simulink model "P_Control"  (R2024b)
settings: Solver=VariableStepAuto  StartTime=0.0  StopTime=time  RelTol=1e-3
values from neighbouring files (symbols this model uses):
  As = 2.15    [Data.m]
  B = (y1-y4)/2    (= 0.75)    [Data.m]
  Cd = 0.28    [Data.m]
  clockwise = 1    [Data.m]
  dd = 2    [Data.m]
  delay_Pulse_time = 1.5    [Data.m]
  derta1 = 0.5    [Data.m]
  dk = 2    [Data.m]
  Fi = Ti/r    (= 156.25)    [Data.m]
  Fz = la/(la+lb)*m*g/2    (= 2450)    [Data.m]
  id = 0.01    [Data.m]
  ik = 1    [Data.m]
  Iw = 0.5    [Data.m]
  Iz = 1600    [Data.m]
  JL = 0.08    [Data.m]
  Jm = 6.96e-6    (= 6.96e-06)    [Data.m]
  Kb = 0.0525    [Data.m]
  Kf = 1.4e-3    (= 0.0014)    [Data.m]
  Km = 0.053    [Data.m]
  L = 6.2e-4    (= 0.00062)    [Data.m]    (also in submit.m = (1-nameda1)*(1-0.015*u1*sqrt((cx^2)*(nameda1^2)+(cy^2)*((tan)
  la = x1    (= 1.25)    [Data.m]
  lb = x1    (= 1.25)    [Data.m]
  m = 1000    [Data.m]
  modeli = 1    [Data.m]
  n = 1/200    (= 0.005)    [Data.m]
  pd = 100    [Data.m]
  pk = 300    [Data.m]
  Pulse = 180    [Data.m]
  R = 2.07    [Data.m]
  r = 0.32    [Data.m]
  s_ang3 = 0    [Data.m]
  x1 = 1.25    [Data.m]
  x1_fc = 0.01    [Data.m]
  x1_jz = 0    [Data.m]
  x2 = -1.25    [Data.m]
  x2_fc = 0.05    [Data.m]
  x2_jz = 0.01    [Data.m]
  x3 = -1.25    [Data.m]
  x3_fc = 0.1    [Data.m]
  x3_jz = 0.05    [Data.m]
  x4 = 1.25    [Data.m]
  x4_fc = 0.5    [Data.m]
  x4_jz = 0.08    [Data.m]
  Xicr = 0,Yicr=10    [Data.m]
  y1 = 0.75    [Data.m]
  y2 = 0.75    [Data.m]
  y3 = -0.75    [Data.m]
  y4 = -0.75    [Data.m]
undefined symbols (not defined in the file or in its folder): Yicr
libraries: slpidlib x12
(part 1 of 2)
settings Model: Creator=hzh  LastModifiedBy=hzh
settings DataIOCC: ReturnWorkspaceOutputsName=out1
settings RTWCC: GPUComputeCapability=3.5

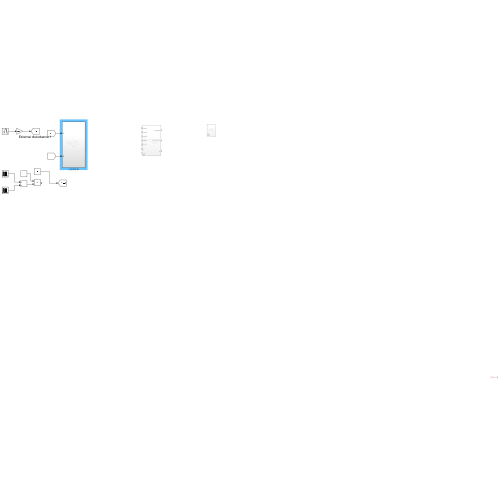
[thumbnail: Simulink's stored preview of the top-level diagram]
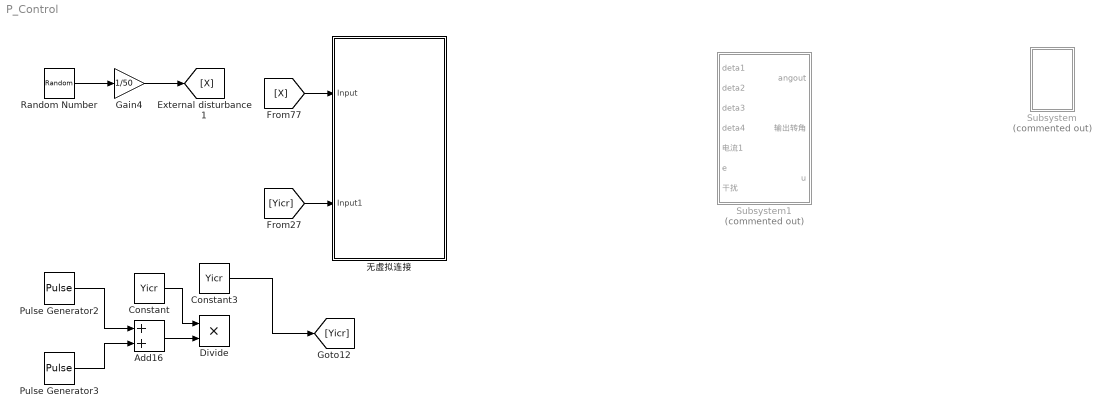
== system P_Control ==
  Add16 : Sum
  Constant : Constant  Value=Yicr
  Constant3 : Constant  Value=Yicr
  Divide : Product  Inputs=**
  Gain4 : Gain  Gain=1/50
  Pulse Generator2 : DiscretePulseGenerator  PulseType=Time based  Period=5  PulseWidth=50
  Pulse Generator3 : DiscretePulseGenerator  PulseType=Time based  Amplitude=-1  Period=5  PulseWidth=50  PhaseDelay=2.5
  Random Number : RandomNumber  SampleTime=0.1
  Subsystem : Subsystem  Commented=on
  Subsystem1 : Subsystem  Commented=on
  无虚拟连接 : Subsystem
  wires:
  ? -> ?
  [Yicr] -> 无虚拟连接/2(Input1)
  [X] -> 无虚拟连接/1(Input)
  Random Number/1 -> Gain4/1
  Gain4/1 -> [X]
  Pulse Generator3/1 -> Add16/2
  Constant/1 -> Divide/1
  Pulse Generator2/1 -> Add16/1
  Add16/1 -> Divide/2
  Constant3/1 -> [Yicr]

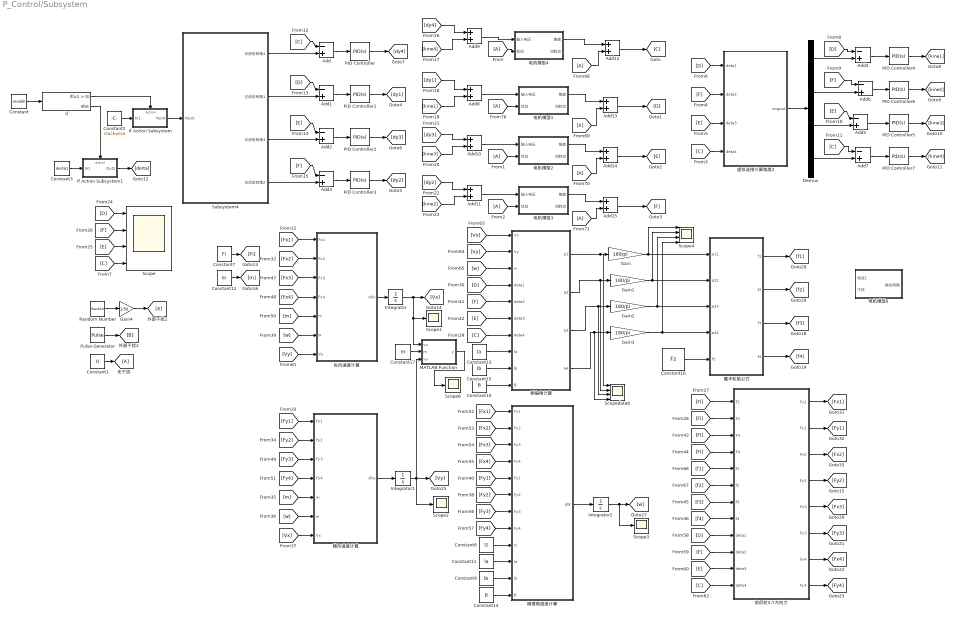
== system P_Control/Subsystem ==
  Add{,1..7} (8 alike) : Sum  Inputs=-+
  Add{8..15} (8 alike) : Sum
  Constant : Constant  Value=modeli
  Constant1 : Constant  Value=0
  Constant10 : Constant  Value=B
  Constant11 : Constant  Value=la
  Constant12 : Constant  Value=m
  Constant13 : Constant  Value=la
  Constant14 : Constant  Value=B
  Constant15 : Constant  Value=lb
  Constant16 : Constant  Value=Fz
  Constant17 : Constant  Value=m
  Constant2 : Constant  Value=clockwise
  Constant3 : Constant  Value=derta1
  Constant7 : Constant  Value=Fi
  Constant8 : Constant  Value=Iz
  Constant9 : Constant  Value=lb
  Demux : Demux
  From{,1..2,68,70..71,76} (7 alike) : From
  Gain{,1..3} (4 alike) : Gain  Gain=180/pi
  Gain4 : Gain  Gain=1/50
  If : If
  If Action Subsystem : Subsystem  TreatAsAtomicUnit=on
  If Action Subsystem1 : Subsystem  TreatAsAtomicUnit=on
  Integrator : Integrator  InitialCondition=0.01
  Integrator1 : Integrator
  Integrator2 : Integrator
  MATLAB Function : MATLAB Function  TreatAsAtomicUnit=on
  PID Controller{,1..3} (4 alike) : slpidlib/PID Controller  Controller=PID  Form=Parallel  TimeDomain=Continuous-time  UseExternalTs=off  SampleTime=-1  IntegratorMethod=Forward Euler  FilterMethod=Forward Euler  ControllerParametersSource=internal  P=pd  I=id  UseKiTs=off  D=dd  N=100  UseFilter=on  TunerSelectOption=Transfer Function Based (PID Tuner App)  InitialConditionSource=internal  InitialConditionForIntegrator=0  InitialConditionForFilter=0  DifferentiatorICPrevScaledInput=0  ExternalReset=none  TrackingMode=off  Kt=1  LimitOutput=off  SatLimitsSource=internal  UpperSaturationLimit=inf  LowerSaturationLimit=-inf  LinearizeAsGain=on  AntiWindupMode=none  Kb=1  LimitIntegrator=off  UpperIntegratorSaturationLimit=inf  LowerIntegratorSaturationLimit=-inf  POutMin=[]  POutMax=[]  IOutMin=[]  IOutMax=[]  DOutMin=[]  DOutMax=[]  NOutMin=[]  NOutMax=[]  SumOutMin=[]  SumOutMax=[]  SaturationOutMin=[]  SaturationOutMax=[]  PParamMin=[]  PParamMax=[]  IParamMin=[]  IParamMax=[]  DParamMin=[]  DParamMax=[]  NParamMin=[]  NParamMax=[]  KbParamMin=[]  KbParamMax=[]  KtParamMin=[]  KtParamMax=[]  KbOutMin=[]  KbOutMax=[]  KtOutMin=[]  KtOutMax=[]  IntegratorOutMin=[]  IntegratorOutMax=[]  FilterOutMin=[]  FilterOutMax=[]  SumI1OutMin=[]  SumI1OutMax=[]  SumI2OutMin=[]  SumI2OutMax=[]  SumI3OutMin=[]  SumI3OutMax=[]  SumI4OutMin=[]  SumI4OutMax=[]  SumDOutMin=[]  SumDOutMax=[]  DifferentiatorOutMin=[]  DifferentiatorOutMax=[]  FilterDiffOutCoefMin=[]  FilterDiffOutCoefMax=[]  ReciprocalOutMin=[]  ReciprocalOutMax=[]  SumDenOutMin=[]  SumDenOutMax=[]  SumNumOutMin=[]  SumNumOutMax=[]  DivideOutMin=[]  DivideOutMax=[]  UdiffTsProdOutMin=[]  UdiffTsProdOutMax=[]  NTsProdOutMin=[]  NTsProdOutMax=[]  UintegralTsProdOutMin=[]  UintegralTsProdOutMax=[]  UngainTsProdOutMin=[]  UngainTsProdOutMax=[]  ClampingZeroOutDataTypeStr=Inherit: Inherit via back propagation  ClampingZeroOutMin=[]  ClampingZeroOutMax=[]  FilterDenConstantOutDataTypeStr=Inherit: Inherit via back propagation  FilterDenConstantOutMin=[]  FilterDenConstantOutMax=[]  PCopyOutDataTypeStr=Inherit: Inherit via back propagation  PCopyOutMin=[]  PCopyOutMax=[]  NCopyOutDataTypeStr=Inherit: Inherit via back propagation  NCopyOutMin=[]  NCopyOutMax=[]  IntegratorContinuousStateAttributes=''  IntegratorStateMustResolveToSignalObject=off  IntegratorRTWStateStorageClass=Auto  FilterContinuousStateAttributes=''  FilterStateMustResolveToSignalObject=off  FilterRTWStateStorageClass=Auto  ParallelPVariant=InternalParameters  IdealPVariant=Disabled  IVariant=InternalParameters  DVariant=InternalParameters  IntegratorVariant=Continuous  SatVariant=Disabled  AWVariant=Passthrough  PCopyVariant=Disabled  TRVariant=Disabled  FdbkBlocksVariant=Forward  IdealPFdbkVariant=Disabled  SatFdbkVariant=Disabled  DerivativeFilterVariant=ContFilter  NVariant=InternalParameters  NCopyVariant=Disabled  FilterICVariant=InternalICsFilter  IntegratorICVariant=InternalICs  ExternalResetVariant=Disabled  TRSumVariant=Passthrough  SumFdbkVariant=Disabled  SumVariant=Sum_PID  TsampFilterVariant=InternalTs  TsampNgainVariant=Passthrough  TsampIntegralVariant=Disabled_SignalSpec  ExternalSaturationOutDataTypeStr=Inherit: Same as second input
  PID Controller4 : slpidlib/PID Controller  Controller=PID  Form=Parallel  TimeDomain=Continuous-time  UseExternalTs=off  SampleTime=-1  IntegratorMethod=Forward Euler  FilterMethod=Forward Euler  ControllerParametersSource=internal  P=pk  I=ik  UseKiTs=off  D=dk  N=100  UseFilter=on  TunerSelectOption=Transfer Function Based (PID Tuner App)  InitialConditionSource=internal  InitialConditionForIntegrator=0  InitialConditionForFilter=0  DifferentiatorICPrevScaledInput=0  ExternalReset=none  TrackingMode=off  Kt=1  LimitOutput=off  SatLimitsSource=internal  UpperSaturationLimit=inf  LowerSaturationLimit=-inf  LinearizeAsGain=on  AntiWindupMode=none  Kb=1  LimitIntegrator=off  UpperIntegratorSaturationLimit=inf  LowerIntegratorSaturationLimit=-inf  POutMin=[]  POutMax=[]  IOutMin=[]  IOutMax=[]  DOutMin=[]  DOutMax=[]  NOutMin=[]  NOutMax=[]  SumOutMin=[]  SumOutMax=[]  SaturationOutMin=[]  SaturationOutMax=[]  PParamMin=[]  PParamMax=[]  IParamMin=[]  IParamMax=[]  DParamMin=[]  DParamMax=[]  NParamMin=[]  NParamMax=[]  KbParamMin=[]  KbParamMax=[]  KtParamMin=[]  KtParamMax=[]  KbOutMin=[]  KbOutMax=[]  KtOutMin=[]  KtOutMax=[]  IntegratorOutMin=[]  IntegratorOutMax=[]  FilterOutMin=[]  FilterOutMax=[]  SumI1OutMin=[]  SumI1OutMax=[]  SumI2OutMin=[]  SumI2OutMax=[]  SumI3OutMin=[]  SumI3OutMax=[]  SumI4OutMin=[]  SumI4OutMax=[]  SumDOutMin=[]  SumDOutMax=[]  DifferentiatorOutMin=[]  DifferentiatorOutMax=[]  FilterDiffOutCoefMin=[]  FilterDiffOutCoefMax=[]  ReciprocalOutMin=[]  ReciprocalOutMax=[]  SumDenOutMin=[]  SumDenOutMax=[]  SumNumOutMin=[]  SumNumOutMax=[]  DivideOutMin=[]  DivideOutMax=[]  UdiffTsProdOutMin=[]  UdiffTsProdOutMax=[]  NTsProdOutMin=[]  NTsProdOutMax=[]  UintegralTsProdOutMin=[]  UintegralTsProdOutMax=[]  UngainTsProdOutMin=[]  UngainTsProdOutMax=[]  ClampingZeroOutDataTypeStr=Inherit: Inherit via back propagation  ClampingZeroOutMin=[]  ClampingZeroOutMax=[]  FilterDenConstantOutDataTypeStr=Inherit: Inherit via back propagation  FilterDenConstantOutMin=[]  FilterDenConstantOutMax=[]  PCopyOutDataTypeStr=Inherit: Inherit via back propagation  PCopyOutMin=[]  PCopyOutMax=[]  NCopyOutDataTypeStr=Inherit: Inherit via back propagation  NCopyOutMin=[]  NCopyOutMax=[]  IntegratorContinuousStateAttributes=''  IntegratorStateMustResolveToSignalObject=off  IntegratorRTWStateStorageClass=Auto  FilterContinuousStateAttributes=''  FilterStateMustResolveToSignalObject=off  FilterRTWStateStorageClass=Auto  ParallelPVariant=InternalParameters  IdealPVariant=Disabled  IVariant=InternalParameters  DVariant=InternalParameters  IntegratorVariant=Continuous  SatVariant=Disabled  AWVariant=Passthrough  PCopyVariant=Disabled  TRVariant=Disabled  FdbkBlocksVariant=Forward  IdealPFdbkVariant=Disabled  SatFdbkVariant=Disabled  DerivativeFilterVariant=ContFilter  NVariant=InternalParameters  NCopyVariant=Disabled  FilterICVariant=InternalICsFilter  IntegratorICVariant=InternalICs  ExternalResetVariant=Disabled  TRSumVariant=Passthrough  SumFdbkVariant=Disabled  SumVariant=Sum_PID  TsampFilterVariant=InternalTs  TsampNgainVariant=Passthrough  TsampIntegralVariant=Disabled_SignalSpec  ExternalSaturationOutDataTypeStr=Inherit: Same as second input
  PID Controller5 : slpidlib/PID Controller  Controller=PID  Form=Parallel  TimeDomain=Continuous-time  UseExternalTs=off  SampleTime=-1  IntegratorMethod=Forward Euler  FilterMethod=Forward Euler  ControllerParametersSource=internal  P=pk  I=ik  UseKiTs=off  D=dk  N=100  UseFilter=on  TunerSelectOption=Frequency Response Based  InitialConditionSource=internal  InitialConditionForIntegrator=0  InitialConditionForFilter=0  DifferentiatorICPrevScaledInput=0  ExternalReset=none  TrackingMode=off  Kt=1  LimitOutput=off  SatLimitsSource=internal  UpperSaturationLimit=inf  LowerSaturationLimit=-inf  LinearizeAsGain=on  AntiWindupMode=none  Kb=1  LimitIntegrator=off  UpperIntegratorSaturationLimit=inf  LowerIntegratorSaturationLimit=-inf  POutMin=[]  POutMax=[]  IOutMin=[]  IOutMax=[]  DOutMin=[]  DOutMax=[]  NOutMin=[]  NOutMax=[]  SumOutMin=[]  SumOutMax=[]  SaturationOutMin=[]  SaturationOutMax=[]  PParamMin=[]  PParamMax=[]  IParamMin=[]  IParamMax=[]  DParamMin=[]  DParamMax=[]  NParamMin=[]  NParamMax=[]  KbParamMin=[]  KbParamMax=[]  KtParamMin=[]  KtParamMax=[]  KbOutMin=[]  KbOutMax=[]  KtOutMin=[]  KtOutMax=[]  IntegratorOutMin=[]  IntegratorOutMax=[]  FilterOutMin=[]  FilterOutMax=[]  SumI1OutMin=[]  SumI1OutMax=[]  SumI2OutMin=[]  SumI2OutMax=[]  SumI3OutMin=[]  SumI3OutMax=[]  SumI4OutMin=[]  SumI4OutMax=[]  SumDOutMin=[]  SumDOutMax=[]  DifferentiatorOutMin=[]  DifferentiatorOutMax=[]  FilterDiffOutCoefMin=[]  FilterDiffOutCoefMax=[]  ReciprocalOutMin=[]  ReciprocalOutMax=[]  SumDenOutMin=[]  SumDenOutMax=[]  SumNumOutMin=[]  SumNumOutMax=[]  DivideOutMin=[]  DivideOutMax=[]  UdiffTsProdOutMin=[]  UdiffTsProdOutMax=[]  NTsProdOutMin=[]  NTsProdOutMax=[]  UintegralTsProdOutMin=[]  UintegralTsProdOutMax=[]  UngainTsProdOutMin=[]  UngainTsProdOutMax=[]  ClampingZeroOutDataTypeStr=Inherit: Inherit via back propagation  ClampingZeroOutMin=[]  ClampingZeroOutMax=[]  FilterDenConstantOutDataTypeStr=Inherit: Inherit via back propagation  FilterDenConstantOutMin=[]  FilterDenConstantOutMax=[]  PCopyOutDataTypeStr=Inherit: Inherit via back propagation  PCopyOutMin=[]  PCopyOutMax=[]  NCopyOutDataTypeStr=Inherit: Inherit via back propagation  NCopyOutMin=[]  NCopyOutMax=[]  IntegratorContinuousStateAttributes=''  IntegratorStateMustResolveToSignalObject=off  IntegratorRTWStateStorageClass=Auto  FilterContinuousStateAttributes=''  FilterStateMustResolveToSignalObject=off  FilterRTWStateStorageClass=Auto  ParallelPVariant=InternalParameters  IdealPVariant=Disabled  IVariant=InternalParameters  DVariant=InternalParameters  IntegratorVariant=Continuous  SatVariant=Disabled  AWVariant=Passthrough  PCopyVariant=Disabled  TRVariant=Disabled  FdbkBlocksVariant=Forward  IdealPFdbkVariant=Disabled  SatFdbkVariant=Disabled  DerivativeFilterVariant=ContFilter  NVariant=InternalParameters  NCopyVariant=Disabled  FilterICVariant=InternalICsFilter  IntegratorICVariant=InternalICs  ExternalResetVariant=Disabled  TRSumVariant=Passthrough  SumFdbkVariant=Disabled  SumVariant=Sum_PID  TsampFilterVariant=InternalTs  TsampNgainVariant=Passthrough  TsampIntegralVariant=Disabled_SignalSpec  ExternalSaturationOutDataTypeStr=Inherit: Same as second input
  PID Controller6 : slpidlib/PID Controller  Controller=PID  Form=Parallel  TimeDomain=Continuous-time  UseExternalTs=off  SampleTime=-1  IntegratorMethod=Forward Euler  FilterMethod=Forward Euler  ControllerParametersSource=internal  P=pk  I=ik  UseKiTs=off  D=dk  N=100  UseFilter=on  TunerSelectOption=Transfer Function Based (PID Tuner App)  InitialConditionSource=internal  InitialConditionForIntegrator=0  InitialConditionForFilter=0  DifferentiatorICPrevScaledInput=0  ExternalReset=none  TrackingMode=off  Kt=1  LimitOutput=off  SatLimitsSource=internal  UpperSaturationLimit=inf  LowerSaturationLimit=-inf  LinearizeAsGain=on  AntiWindupMode=none  Kb=1  LimitIntegrator=off  UpperIntegratorSaturationLimit=inf  LowerIntegratorSaturationLimit=-inf  POutMin=[]  POutMax=[]  IOutMin=[]  IOutMax=[]  DOutMin=[]  DOutMax=[]  NOutMin=[]  NOutMax=[]  SumOutMin=[]  SumOutMax=[]  SaturationOutMin=[]  SaturationOutMax=[]  PParamMin=[]  PParamMax=[]  IParamMin=[]  IParamMax=[]  DParamMin=[]  DParamMax=[]  NParamMin=[]  NParamMax=[]  KbParamMin=[]  KbParamMax=[]  KtParamMin=[]  KtParamMax=[]  KbOutMin=[]  KbOutMax=[]  KtOutMin=[]  KtOutMax=[]  IntegratorOutMin=[]  IntegratorOutMax=[]  FilterOutMin=[]  FilterOutMax=[]  SumI1OutMin=[]  SumI1OutMax=[]  SumI2OutMin=[]  SumI2OutMax=[]  SumI3OutMin=[]  SumI3OutMax=[]  SumI4OutMin=[]  SumI4OutMax=[]  SumDOutMin=[]  SumDOutMax=[]  DifferentiatorOutMin=[]  DifferentiatorOutMax=[]  FilterDiffOutCoefMin=[]  FilterDiffOutCoefMax=[]  ReciprocalOutMin=[]  ReciprocalOutMax=[]  SumDenOutMin=[]  SumDenOutMax=[]  SumNumOutMin=[]  SumNumOutMax=[]  DivideOutMin=[]  DivideOutMax=[]  UdiffTsProdOutMin=[]  UdiffTsProdOutMax=[]  NTsProdOutMin=[]  NTsProdOutMax=[]  UintegralTsProdOutMin=[]  UintegralTsProdOutMax=[]  UngainTsProdOutMin=[]  UngainTsProdOutMax=[]  ClampingZeroOutDataTypeStr=Inherit: Inherit via back propagation  ClampingZeroOutMin=[]  ClampingZeroOutMax=[]  FilterDenConstantOutDataTypeStr=Inherit: Inherit via back propagation  FilterDenConstantOutMin=[]  FilterDenConstantOutMax=[]  PCopyOutDataTypeStr=Inherit: Inherit via back propagation  PCopyOutMin=[]  PCopyOutMax=[]  NCopyOutDataTypeStr=Inherit: Inherit via back propagation  NCopyOutMin=[]  NCopyOutMax=[]  IntegratorContinuousStateAttributes=''  IntegratorStateMustResolveToSignalObject=off  IntegratorRTWStateStorageClass=Auto  FilterContinuousStateAttributes=''  FilterStateMustResolveToSignalObject=off  FilterRTWStateStorageClass=Auto  ParallelPVariant=InternalParameters  IdealPVariant=Disabled  IVariant=InternalParameters  DVariant=InternalParameters  IntegratorVariant=Continuous  SatVariant=Disabled  AWVariant=Passthrough  PCopyVariant=Disabled  TRVariant=Disabled  FdbkBlocksVariant=Forward  IdealPFdbkVariant=Disabled  SatFdbkVariant=Disabled  DerivativeFilterVariant=ContFilter  NVariant=InternalParameters  NCopyVariant=Disabled  FilterICVariant=InternalICsFilter  IntegratorICVariant=InternalICs  ExternalResetVariant=Disabled  TRSumVariant=Passthrough  SumFdbkVariant=Disabled  SumVariant=Sum_PID  TsampFilterVariant=InternalTs  TsampNgainVariant=Passthrough  TsampIntegralVariant=Disabled_SignalSpec  ExternalSaturationOutDataTypeStr=Inherit: Same as second input
  PID Controller7 : slpidlib/PID Controller  Controller=PID  Form=Parallel  TimeDomain=Continuous-time  UseExternalTs=off  SampleTime=-1  IntegratorMethod=Forward Euler  FilterMethod=Forward Euler  ControllerParametersSource=internal  P=pk  I=ik  UseKiTs=off  D=dk  N=100  UseFilter=on  TunerSelectOption=Transfer Function Based (PID Tuner App)  InitialConditionSource=internal  InitialConditionForIntegrator=0  InitialConditionForFilter=0  DifferentiatorICPrevScaledInput=0  ExternalReset=none  TrackingMode=off  Kt=1  LimitOutput=off  SatLimitsSource=internal  UpperSaturationLimit=inf  LowerSaturationLimit=-inf  LinearizeAsGain=on  AntiWindupMode=none  Kb=1  LimitIntegrator=off  UpperIntegratorSaturationLimit=inf  LowerIntegratorSaturationLimit=-inf  POutMin=[]  POutMax=[]  IOutMin=[]  IOutMax=[]  DOutMin=[]  DOutMax=[]  NOutMin=[]  NOutMax=[]  SumOutMin=[]  SumOutMax=[]  SaturationOutMin=[]  SaturationOutMax=[]  PParamMin=[]  PParamMax=[]  IParamMin=[]  IParamMax=[]  DParamMin=[]  DParamMax=[]  NParamMin=[]  NParamMax=[]  KbParamMin=[]  KbParamMax=[]  KtParamMin=[]  KtParamMax=[]  KbOutMin=[]  KbOutMax=[]  KtOutMin=[]  KtOutMax=[]  IntegratorOutMin=[]  IntegratorOutMax=[]  FilterOutMin=[]  FilterOutMax=[]  SumI1OutMin=[]  SumI1OutMax=[]  SumI2OutMin=[]  SumI2OutMax=[]  SumI3OutMin=[]  SumI3OutMax=[]  SumI4OutMin=[]  SumI4OutMax=[]  SumDOutMin=[]  SumDOutMax=[]  DifferentiatorOutMin=[]  DifferentiatorOutMax=[]  FilterDiffOutCoefMin=[]  FilterDiffOutCoefMax=[]  ReciprocalOutMin=[]  ReciprocalOutMax=[]  SumDenOutMin=[]  SumDenOutMax=[]  SumNumOutMin=[]  SumNumOutMax=[]  DivideOutMin=[]  DivideOutMax=[]  UdiffTsProdOutMin=[]  UdiffTsProdOutMax=[]  NTsProdOutMin=[]  NTsProdOutMax=[]  UintegralTsProdOutMin=[]  UintegralTsProdOutMax=[]  UngainTsProdOutMin=[]  UngainTsProdOutMax=[]  ClampingZeroOutDataTypeStr=Inherit: Inherit via back propagation  ClampingZeroOutMin=[]  ClampingZeroOutMax=[]  FilterDenConstantOutDataTypeStr=Inherit: Inherit via back propagation  FilterDenConstantOutMin=[]  FilterDenConstantOutMax=[]  PCopyOutDataTypeStr=Inherit: Inherit via back propagation  PCopyOutMin=[]  PCopyOutMax=[]  NCopyOutDataTypeStr=Inherit: Inherit via back propagation  NCopyOutMin=[]  NCopyOutMax=[]  IntegratorContinuousStateAttributes=''  IntegratorStateMustResolveToSignalObject=off  IntegratorRTWStateStorageClass=Auto  FilterContinuousStateAttributes=''  FilterStateMustResolveToSignalObject=off  FilterRTWStateStorageClass=Auto  ParallelPVariant=InternalParameters  IdealPVariant=Disabled  IVariant=InternalParameters  DVariant=InternalParameters  IntegratorVariant=Continuous  SatVariant=Disabled  AWVariant=Passthrough  PCopyVariant=Disabled  TRVariant=Disabled  FdbkBlocksVariant=Forward  IdealPFdbkVariant=Disabled  SatFdbkVariant=Disabled  DerivativeFilterVariant=ContFilter  NVariant=InternalParameters  NCopyVariant=Disabled  FilterICVariant=InternalICsFilter  IntegratorICVariant=InternalICs  ExternalResetVariant=Disabled  TRSumVariant=Passthrough  SumFdbkVariant=Disabled  SumVariant=Sum_PID  TsampFilterVariant=InternalTs  TsampNgainVariant=Passthrough  TsampIntegralVariant=Disabled_SignalSpec  ExternalSaturationOutDataTypeStr=Inherit: Same as second input
  Pulse Generator : DiscretePulseGenerator  PulseType=Time based  Amplitude=Pulse  Period=100  PulseWidth=0.2  PhaseDelay=delay_Pulse_time
  Random Number : RandomNumber  SampleTime=0.1
  Scope : Scope  NumInputPorts=4
  Scope{1..3,6} (4 alike) : Scope
  Scope4 : Scope  NumInputPorts=4
  Scopedata6 : Scope  NumInputPorts=4
  Subsystem4 : Subsystem
  侧偏角计算 : MATLAB Function  TreatAsAtomicUnit=on
  前后轮X,Y方向力 : MATLAB Function  TreatAsAtomicUnit=on
  无干扰 : Goto
  横向速度计算 : MATLAB Function  TreatAsAtomicUnit=on
  横摆角速度计算 : MATLAB Function  TreatAsAtomicUnit=on
  电机模型1 : Subsystem
  电机模型2 : Subsystem
  电机模型3 : Subsystem
  电机模型4 : Subsystem
  电机模型6 : Subsystem
  纵向速度计算 : MATLAB Function  TreatAsAtomicUnit=on
  虚拟连接计算角度2 : MATLAB Function  TreatAsAtomicUnit=on
  魔术轮胎公式 : MATLAB Function  TreatAsAtomicUnit=on
  wires:
  [C] -> 前后轮X,Y方向力/12(deta4)
  Add2/1 -> PID Controller2/1
  MATLAB Function/1(y) -> Scope6/1
  前后轮X,Y方向力/2(Fy1) -> [Fy1]
  Add12/1 -> [C]
  [w] -> 横向速度计算/6(w)
  [D] -> 侧偏角计算/4(deta1)
  Integrator/1 -> [Vx], MATLAB Function/1(vx), Scope1/1
  PID Controller/1 -> [dy4]
  虚拟连接计算角度2/1(angout) -> Demux/1
  [Fy4] -> 横向速度计算/4(Fy4)
  [Fx1] -> 横摆角速度计算/1(Fx1)
  [m] -> 横向速度计算/5(m)
  [kine4] -> Add9/2
  Add6/1 -> PID Controller6/1
  PID Controller4/1 -> [kine1]
  Add14/1 -> [E]
  前后轮X,Y方向力/3(Fx2) -> [Fx2]
  [f2] -> 前后轮X,Y方向力/6(f2)
  If/1 -> If Action Subsystem/Action
  Gain4/1 -> [X]
  Add11/1 -> 电机模型3/1(输入电压)
  [Fx4] -> 横摆角速度计算/4(Fx4)
  [Fx2] -> 纵向速度计算/2(Fx2)
  Constant16/1 -> 魔术轮胎公式/5(Fz)
  PID Controller2/1 -> [dy3]
  From2/1 -> 电机模型3/2(扰动)
  Demux/2 -> Add6/2
  If/2 -> If Action Subsystem1/Action
  From76/1 -> 电机模型1/2(扰动)
  [Fy2] -> 横向速度计算/2(Fy2)
  Random Number/1 -> Gain4/1
  [Vy] -> 侧偏角计算/2(Vy)
  Gain3/1 -> Scope4/4, 魔术轮胎公式/4(a44)
  [m] -> 纵向速度计算/5(m)
  If Action Subsystem1/1(Out1) -> [derta]
  Constant2/1 -> If Action Subsystem/1(In1)
  Constant12/1 -> [m]
  魔术轮胎公式/1(f1) -> [f1]
  From71/1 -> Add15/2
  Add15/1 -> [F]
  If Action Subsystem/1(Input) -> Subsystem4/1(Input)
  [D] -> 前后轮X,Y方向力/9(deta1)
  Add1/1 -> PID Controller1/1
  PID Controller6/1 -> [kine2]
  PID Controller3/1 -> [dy2]
  [w] -> 侧偏角计算/3(w)
  [E] -> 侧偏角计算/6(deta3)
  Constant10/1 -> 侧偏角计算/10(B)
  From1/1 -> 电机模型2/2(扰动)
  [Fy1] -> 横向速度计算/1(Fy1)
  Add10/1 -> 电机模型2/1(输入电压)
  [C] -> 侧偏角计算/7(deta4)
  Subsystem4/4(左后轮转角2) -> Add3/2
  [F] -> 虚拟连接计算角度2/2(deta2)
  [C] -> 虚拟连接计算角度2/4(deta4)
  魔术轮胎公式/2(f2) -> [f2]
  Subsystem4/3(右后轮转角3) -> Add2/2
  Integrator2/1 -> Scope3/1, [w]
  纵向速度计算/1(dVx) -> Integrator/1
  魔术轮胎公式/4(f4) -> [f4]
  [Fi] -> 前后轮X,Y方向力/1(F1)
  [Fi] -> 前后轮X,Y方向力/3(F3)
  [dy2] -> Add11/1
  Demux/1 -> Add4/2
  [C] -> Add/1
  横摆角速度计算/1(dW) -> Integrator2/1
  Demux/3 -> Add5/2
  [X] -> Add13/2
  Add13/1 -> [D]
  Subsystem4/2(左前轮转角1) -> Add1/2
  From68/1 -> Add12/2
  Subsystem4/1(右前轮转角4) -> Add/2
  Constant1/1 -> 无干扰/1
  [dy4] -> Add9/1
  [dy1] -> Add8/1
  From70/1 -> Add14/2
  Add5/1 -> PID Controller5/1
  PID Controller5/1 -> [kine3]
  [D] -> Scope/1
  Add7/1 -> PID Controller7/1
  Add3/1 -> PID Controller3/1
  [F] -> Add3/1
  [E] -> Add2/1
  [E] -> 虚拟连接计算角度2/3(deta3)
  [D] -> Add1/1
  PID Controller1/1 -> [dy1]
  [D] -> Add4/1
  Constant17/1 -> MATLAB Function/2(m)
  Add/1 -> PID Controller/1
  [Fx3] -> 纵向速度计算/3(Fx3)
  [kine3] -> Add10/2
  侧偏角计算/4(a4) -> Scopedata6/4, Gain3/1
  Constant11/1 -> 横摆角速度计算/10(la)
  Add4/1 -> PID Controller4/1
  侧偏角计算/3(a3) -> Scopedata6/3, Gain2/1
  [Fy4] -> 横摆角速度计算/8(Fy4)
  [E] -> 前后轮X,Y方向力/11(deta3)
  Integrator1/1 -> MATLAB Function/3(vy), Scope2/1, [Vy]
  [E] -> Add5/1
  前后轮X,Y方向力/5(Fx3) -> [Fx3]
  前后轮X,Y方向力/4(Fy2) -> [Fy2]
  Gain1/1 -> Scope4/2, 魔术轮胎公式/2(a22)
  Constant9/1 -> 横摆角速度计算/11(lb)
  [f1] -> 前后轮X,Y方向力/5(f1)
  [dy3] -> Add10/1
  [Fx3] -> 横摆角速度计算/3(Fx3)
  前后轮X,Y方向力/7(Fx4) -> [Fx4]
  Demux/4 -> Add7/2
  Constant13/1 -> 侧偏角计算/8(la)
  [Fy1] -> 横摆角速度计算/5(Fy1)
  [kine1] -> Add8/2
  Constant/1 -> If/1
  侧偏角计算/2(a2) -> Scopedata6/2, Gain1/1
  [w] -> 纵向速度计算/6(w)
  [Fx2] -> 横摆角速度计算/2(Fx2)
  [Fy2] -> 横摆角速度计算/6(Fy2)
  前后轮X,Y方向力/1(Fx1) -> [Fx1]
  Constant15/1 -> 侧偏角计算/9(lb)
  侧偏角计算/1(a1) -> Scopedata6/1, Gain/1
  Constant3/1 -> If Action Subsystem1/1(In1)
  横向速度计算/1(dVy) -> Integrator1/1
  Gain2/1 -> Scope4/3, 魔术轮胎公式/3(a33)
  前后轮X,Y方向力/8(Fy4) -> [Fy4]
  [F] -> Add6/1
  [E] -> Scope/3
  前后轮X,Y方向力/6(Fy3) -> [Fy3]
  [Vy] -> 纵向速度计算/7(Vy)
  [Fi] -> 前后轮X,Y方向力/4(F4)
  [Fy3] -> 横摆角速度计算/7(Fy3)
  Pulse Generator/1 -> [B]
  [C] -> Scope/4
  [f3] -> 前后轮X,Y方向力/7(f3)
  Constant8/1 -> 横摆角速度计算/9(Iz)
  [D] -> 虚拟连接计算角度2/1(deta1)
  Constant7/1 -> [Fi]
  [F] -> 侧偏角计算/5(deta2)
  Add8/1 -> 电机模型1/1(输入电压)
  [C] -> Add7/1
  [F] -> Scope/2
  Constant14/1 -> 横摆角速度计算/12(B)
  [Fy3] -> 横向速度计算/3(Fy3)
  [Fx4] -> 纵向速度计算/4(Fx4)
  [Vx] -> 侧偏角计算/1(Vx)
  [F] -> 前后轮X,Y方向力/10(deta2)
  [f4] -> 前后轮X,Y方向力/8(f4)
  [kine2] -> Add11/2
  [Fi] -> 前后轮X,Y方向力/2(F2)
  [Vx] -> 横向速度计算/7(Vx)
  魔术轮胎公式/3(f3) -> [f3]
  PID Controller7/1 -> [kine4]
  Gain/1 -> Scope4/1, 魔术轮胎公式/1(a11)
  [Fx1] -> 纵向速度计算/1(Fx1)
  Add9/1 -> 电机模型4/1(输入电压)
  From/1 -> 电机模型4/2(扰动)
  电机模型4/1(角度) -> Add12/1
  电机模型2/1(角度) -> Add14/1
  电机模型3/1(角度) -> Add15/1
  电机模型1/1(角度) -> Add13/1

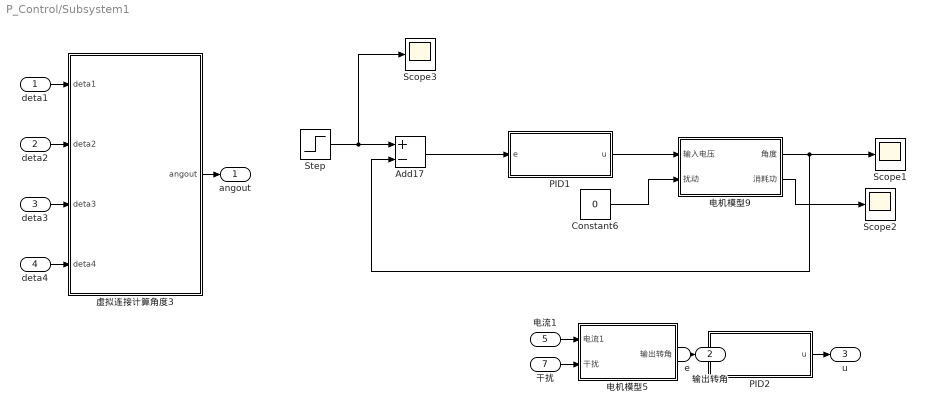
== system P_Control/Subsystem1 ==
  deta1 : Inport
  deta2 : Inport  Port=2
  deta3 : Inport  Port=3
  deta4 : Inport  Port=4
  电流1 : Inport  Port=5
  e : Inport  Port=6
  干扰 : Inport  Port=7
  Add17 : Sum  Inputs=+-
  Constant6 : Constant  Value=0
  PID1 : Subsystem
  PID2 : Subsystem
  Scope1 : Scope
  Scope2 : Scope
  Scope3 : Scope
  Step : Step  SampleTime=0
  电机模型5 : Subsystem
  电机模型9 : Subsystem
  虚拟连接计算角度3 : MATLAB Function  TreatAsAtomicUnit=on
  angout : Outport
  输出转角 : Outport  Port=2
  u : Outport  Port=3
  wires:
  电流1/1 -> 电机模型5/1(电流1)
  Step/1 -> Scope3/1, Add17/1
  PID1/1(u) -> 电机模型9/1(输入电压)
  Constant6/1 -> 电机模型9/2(扰动)
  电机模型9/1(角度) -> Scope1/1, Add17/2
  Add17/1 -> PID1/1(e)
  deta4/1 -> 虚拟连接计算角度3/4(deta4)
  电机模型9/2(消耗功) -> Scope2/1
  虚拟连接计算角度3/1(angout) -> angout/1
  干扰/1 -> 电机模型5/2(干扰)
  deta2/1 -> 虚拟连接计算角度3/2(deta2)
  电机模型5/1(输出转角) -> 输出转角/1
  deta1/1 -> 虚拟连接计算角度3/1(deta1)
  deta3/1 -> 虚拟连接计算角度3/3(deta3)
  PID2/1(u) -> u/1
  e/1 -> PID2/1(e)

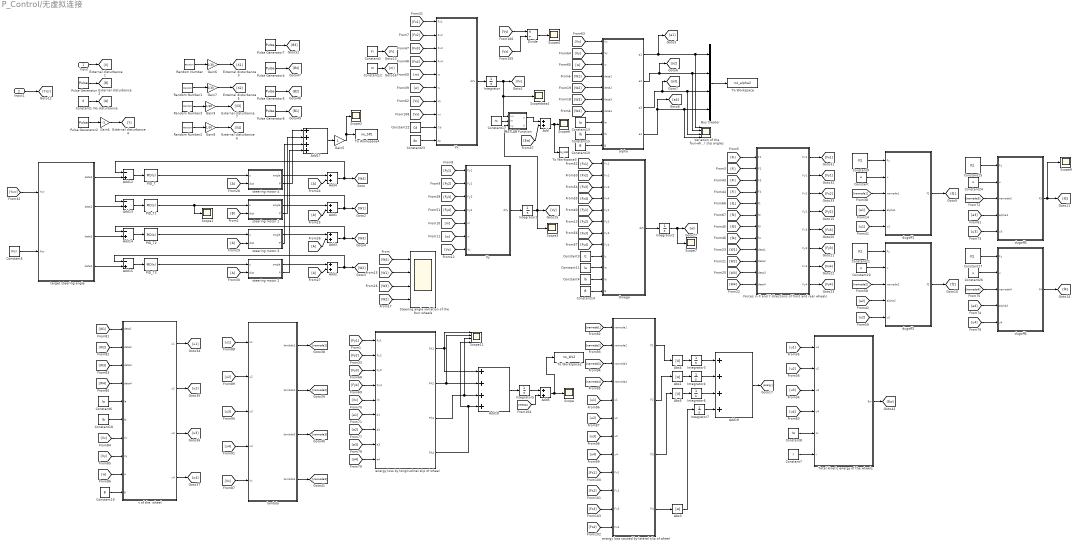
== system P_Control/无虚拟连接 ==
  Input : Inport
  Input1 : Inport  Port=2
  " target steering angle" : MATLAB Function  TreatAsAtomicUnit=on
  Abs{1,3..5} (4 alike) : Abs  SaturateOnIntegerOverflow=off
  Add{,1..5} (6 alike) : Sum
  Add{12..15} (4 alike) : Sum  Inputs=-+
  Add17 : Sum  Inputs=++++
  Add18 : Sum  Inputs=++++
  Add19 : Sum  Inputs=++++
  Bus Creator : BusCreator  Inputs=4
  Constant{,20,24,26} (4 alike) : Constant  Value=u
  Constant1 : Constant  Value=0
  Constant10 : Constant  Value=B
  Constant11 : Constant  Value=la
  Constant12 : Constant  Value=m
  Constant13 : Constant  Value=la
  Constant14 : Constant  Value=B
  Constant15 : Constant  Value=lb
  Constant17 : Constant  Value=m
  Constant18 : Constant  Value=lb
  Constant19 : Constant  Value=B
  Constant2 : Constant  Value=Fi
  Constant{9,21,25,27} (4 alike) : Constant  Value=Fz
  Constant22 : Constant  Value=Cd
  Constant23 : Constant  Value=As
  Constant3 : Constant  Value=Iz
  Constant4 : Constant  Value=lb
  Constant5 : Constant  Value=Xicr
  Constant6 : Constant  Value=la
  Constant7 : Constant  Value=r
  Constant8 : Constant  Value=Iw
  Divide : Product  Inputs=*/
  Forces in X and Y directions of front and rear wheels : MATLAB Function  TreatAsAtomicUnit=on
  From{24..30} (7 alike) : From
  Gain4 : Gain  Gain=-1
  Gain5 : Gain
  Gain{6..9} (4 alike) : Gain  Gain=1/30
  Integrator : Integrator  InitialCondition=0.0001
  Integrator1 : Integrator
  Integrator2 : Integrator
  Integrator{3..7} (5 alike) : Integrator  InitialCondition=0.01
  MATLAB Function : MATLAB Function  TreatAsAtomicUnit=on
  No disturbance : Goto
  Omega : MATLAB Function  TreatAsAtomicUnit=on
  PID_T{,1..3} (4 alike) : slpidlib/PID Controller  Controller=PID  Form=Parallel  TimeDomain=Continuous-time  UseExternalTs=off  SampleTime=-1  IntegratorMethod=Forward Euler  FilterMethod=Forward Euler  ControllerParametersSource=internal  P=pd  I=id  UseKiTs=off  D=dd  UseExternalDerivativeSource=off  N=100  UseFilter=on  TunerSelectOption=Transfer Function Based (PID Tuner App)  InitialConditionSource=internal  InitialConditionForIntegrator=0  InitialConditionForFilter=0  DifferentiatorICPrevScaledInput=0  ExternalReset=none  TrackingMode=off  Kt=1  LimitOutput=off  SatLimitsSource=internal  UpperSaturationLimit=inf  LowerSaturationLimit=-inf  LinearizeAsGain=on  AntiWindupMode=none  Kb=1  LimitIntegrator=off  UpperIntegratorSaturationLimit=inf  LowerIntegratorSaturationLimit=-inf  POutMin=[]  POutMax=[]  IOutMin=[]  IOutMax=[]  DOutMin=[]  DOutMax=[]  NOutMin=[]  NOutMax=[]  SumOutMin=[]  SumOutMax=[]  SaturationOutMin=[]  SaturationOutMax=[]  PParamMin=[]  PParamMax=[]  IParamMin=[]  IParamMax=[]  DParamMin=[]  DParamMax=[]  NParamMin=[]  NParamMax=[]  KbParamMin=[]  KbParamMax=[]  KtParamMin=[]  KtParamMax=[]  KbOutMin=[]  KbOutMax=[]  KtOutMin=[]  KtOutMax=[]  IntegratorOutMin=[]  IntegratorOutMax=[]  FilterOutMin=[]  FilterOutMax=[]  SumI1OutMin=[]  SumI1OutMax=[]  SumI2OutMin=[]  SumI2OutMax=[]  SumI3OutMin=[]  SumI3OutMax=[]  SumI4OutMin=[]  SumI4OutMax=[]  SumDOutMin=[]  SumDOutMax=[]  DifferentiatorOutMin=[]  DifferentiatorOutMax=[]  FilterDiffOutCoefMin=[]  FilterDiffOutCoefMax=[]  ReciprocalOutMin=[]  ReciprocalOutMax=[]  SumDenOutMin=[]  SumDenOutMax=[]  SumNumOutMin=[]  SumNumOutMax=[]  DivideOutMin=[]  DivideOutMax=[]  UdiffTsProdOutMin=[]  UdiffTsProdOutMax=[]  NTsProdOutMin=[]  NTsProdOutMax=[]  UintegralTsProdOutMin=[]  UintegralTsProdOutMax=[]  UngainTsProdOutMin=[]  UngainTsProdOutMax=[]  ClampingZeroOutDataTypeStr=Inherit: Inherit via back propagation  ClampingZeroOutMin=[]  ClampingZeroOutMax=[]  FilterDenConstantOutDataTypeStr=Inherit: Inherit via back propagation  FilterDenConstantOutMin=[]  FilterDenConstantOutMax=[]  PCopyOutDataTypeStr=Inherit: Inherit via back propagation  PCopyOutMin=[]  PCopyOutMax=[]  NCopyOutDataTypeStr=Inherit: Inherit via back propagation  NCopyOutMin=[]  NCopyOutMax=[]  IntegratorContinuousStateAttributes=''  IntegratorStateMustResolveToSignalObject=off  IntegratorRTWStateStorageClass=Auto  FilterContinuousStateAttributes=''  FilterStateMustResolveToSignalObject=off  FilterRTWStateStorageClass=Auto  ParallelPVariant=InternalParameters  IdealPVariant=Disabled  IVariant=InternalParameters  DVariant=InternalParameters  IntegratorVariant=Continuous  SatVariant=Disabled  AWVariant=Passthrough  PCopyVariant=Disabled  TRVariant=Disabled  FdbkBlocksVariant=Forward  IdealPFdbkVariant=Disabled  SatFdbkVariant=Disabled  DerivativeFilterVariant=ContFilter  NVariant=InternalParameters  NCopyVariant=Disabled  FilterICVariant=InternalICsFilter  IntegratorICVariant=InternalICs  ExternalResetVariant=Disabled  TRSumVariant=Passthrough  SumFdbkVariant=Disabled  SumVariant=Sum_PID  TsampFilterVariant=InternalTs  TsampNgainVariant=Passthrough  TsampIntegralVariant=Disabled_SignalSpec  ExternalSaturationOutDataTypeStr=Inherit: Same as second input  DerivativeSourceVariant=ErrorSignal  PreIntVariant=InternalPreInt
  Pulse Generator : DiscretePulseGenerator  PulseType=Time based  Amplitude=Pulse  Period=100  PulseWidth=0.2  PhaseDelay=delay_Pulse_time
  Pulse Generator2 : DiscretePulseGenerator  PulseType=Time based  Amplitude=Pulse  Period=100  PulseWidth=0.2  PhaseDelay=delay_Pulse_time
  Pulse Generator4 : DiscretePulseGenerator  PulseType=Time based  Amplitude=0.16  Period=15  PulseWidth=15  PhaseDelay=12
  Pulse Generator5 : DiscretePulseGenerator  PulseType=Time based  Amplitude=0.1  Period=15  PulseWidth=5  PhaseDelay=8
  Pulse Generator6 : DiscretePulseGenerator  PulseType=Time based  Amplitude=0.05  Period=10  PulseWidth=5  PhaseDelay=4
  Pulse Generator7 : DiscretePulseGenerator  PulseType=Time based  Amplitude=0.2  Period=15  PulseWidth=4  PhaseDelay=1.5
  Random Number : RandomNumber  Mean=x1_jz  Variance=x1_fc  SampleTime=0.1
  Random Number1 : RandomNumber  Mean=x2_jz  Variance=x2_fc  SampleTime=0.1
  Random Number2 : RandomNumber  Mean=x4_jz  Variance=x4_fc  SampleTime=0.1
  Random Number3 : RandomNumber  Mean=x3_jz  Variance=x3_fc  SampleTime=0.1
  Scope{,1..4,6..7,9} (8 alike) : Scope
  Scope11 : Scope  NumInputPorts=4
  Scopedata4 : Scope
  Steering angle variation of the four wheels : Scope  NumInputPorts=4
  To Workspace : ToWorkspace  VariableName=no_alpha2  SampleTime=-1
  To Workspace2 : ToWorkspace  VariableName=no_WL2  SampleTime=-1
  To Workspace3 : ToWorkspace  VariableName=no_KE2  SampleTime=-1
  To Workspace4 : ToWorkspace  VariableName=no_SP2  SampleTime=-1
  Total kinetic energy of the wheels : MATLAB Function  TreatAsAtomicUnit=on
  Variation of the four-wheel slip angles : Scope  NumInputPorts=4
  Vx : MATLAB Function  TreatAsAtomicUnit=on
  Vy : MATLAB Function  TreatAsAtomicUnit=on
  alpha : MATLAB Function  TreatAsAtomicUnit=on
  "dugoff1 " : MATLAB Function  TreatAsAtomicUnit=on
  dugoff2 : MATLAB Function  TreatAsAtomicUnit=on
  dugoff3 : MATLAB Function  TreatAsAtomicUnit=on
  dugoff4 : MATLAB Function  TreatAsAtomicUnit=on
  energy loss by longitudinal slip of wheel : MATLAB Function  TreatAsAtomicUnit=on
  energy loss caused by lateral slip of wheel : MATLAB Function  TreatAsAtomicUnit=on
  lambda : MATLAB Function  TreatAsAtomicUnit=on
  steering motor 1 : Subsystem
  steering motor 2 : Subsystem
  steering motor 3 : Subsystem
  steering motor 4 : Subsystem
  v of the  wheel : MATLAB Function  TreatAsAtomicUnit=on
  wires:
  From30/1 -> steering motor 2/2(dist)
  Add12/1 -> PID_T/1
  steering motor 3/1(angle) -> Add3/1
  From29/1 -> steering motor 3/2(dist)
  Add14/1 -> PID_T2/1
  PID_T2/1 -> steering motor 3/1(u)
  PID_T1/1 -> Scope1/1, steering motor 1/1(u)
  Add13/1 -> PID_T1/1
  steering motor 1/1(angle) -> Add1/1
  PID_T3/1 -> steering motor 2/1(u)
  [B] -> steering motor 1/2(dist)
  Add15/1 -> PID_T3/1
  From28/1 -> steering motor 4/2(dist)
  Constant1/1 -> No disturbance/1
  Forces in X and Y directions of front and rear wheels/3(Fx2) -> [Fx2]
  Constant10/1 -> alpha/10(B)
  [Fy3] -> Omega/7(Fy3)
  alpha/3(a3) -> [a3], Bus Creator/3, Variation of the four-wheel slip angles/3
  [W1] -> alpha/4(deta1)
  Constant15/1 -> alpha/9(lb)
  [Fi] -> Forces in X and Y directions of front and rear wheels/3(F3)
  [Fy4] -> Omega/8(Fy4)
  [W4] -> Forces in X and Y directions of front and rear wheels/12(deta4)
  [Fy3] -> Vy/3(Fy3)
  [Fx1] -> Omega/1(Fx1)
  Constant11/1 -> Omega/10(la)
  [Fy1] -> Omega/5(Fy1)
  Forces in X and Y directions of front and rear wheels/6(Fy3) -> [Fy3]
  [Fx2] -> Omega/2(Fx2)
  [Fi] -> Forces in X and Y directions of front and rear wheels/2(F2)
  [W4] -> alpha/7(deta4)
  [w] -> alpha/3(w)
  Forces in X and Y directions of front and rear wheels/4(Fy2) -> [Fy2]
  Forces in X and Y directions of front and rear wheels/1(Fx1) -> [Fx1]
  [Fy2] -> Vy/2(Fy2)
  Constant3/1 -> Omega/9(Iz)
  [Fx4] -> Omega/4(Fx4)
  [Fi] -> Forces in X and Y directions of front and rear wheels/4(F4)
  [Fy4] -> Vy/4(Fy4)
  [f3] -> Forces in X and Y directions of front and rear wheels/7(f3)
  [Fy2] -> Omega/6(Fy2)
  Constant13/1 -> alpha/8(la)
  Constant4/1 -> Omega/11(lb)
  Constant14/1 -> Omega/12(B)
  [f4] -> Forces in X and Y directions of front and rear wheels/8(f4)
  Integrator/1 -> [Vx], Scopedata4/1, MATLAB Function/1(vx)
  Omega/1(dW) -> Integrator2/1
  [Fx3] -> Omega/3(Fx3)
  [Fy1] -> Vy/1(Fy1)
  alpha/2(a2) -> [a2], Bus Creator/2, Variation of the four-wheel slip angles/2
  Constant2/1 -> [Fi]
  [W3] -> Forces in X and Y directions of front and rear wheels/11(deta3)
  Forces in X and Y directions of front and rear wheels/7(Fx4) -> [Fx4]
  [Vy] -> alpha/2(Vy)
  [W3] -> alpha/6(deta3)
  [W2] -> alpha/5(deta2)
  [f2] -> Forces in X and Y directions of front and rear wheels/6(f2)
  Forces in X and Y directions of front and rear wheels/8(Fy4) -> [Fy4]
  Integrator1/1 -> MATLAB Function/3(vy), Scope3/1, [Vy]
  Constant12/1 -> [m]
  Forces in X and Y directions of front and rear wheels/5(Fx3) -> [Fx3]
  Vx/1(dVx) -> Integrator/1
  [Vx] -> alpha/1(Vx)
  [f1] -> Forces in X and Y directions of front and rear wheels/5(f1)
  [W2] -> Forces in X and Y directions of front and rear wheels/10(deta2)
  Integrator2/1 -> Scope7/1, [w]
  [Fi] -> Forces in X and Y directions of front and rear wheels/1(F1)
  [W1] -> Forces in X and Y directions of front and rear wheels/9(deta1)
  Forces in X and Y directions of front and rear wheels/2(Fy1) -> [Fy1]
  Vy/1(dVy) -> Integrator1/1
  [w] -> Vy/6(w)
  [Vx] -> Vy/7(Vx)
  [m] -> Vy/5(m)
  [W4] -> Steering angle variation of the four wheels/1
  [W1] -> Steering angle variation of the four wheels/2
  [W3] -> Steering angle variation of the four wheels/3
  [W2] -> Steering angle variation of the four wheels/4
  PID_T/1 -> steering motor 4/1(u)
  Constant17/1 -> MATLAB Function/2(m)
  Input/1 -> [X]
  Add4/1 -> Add12/1, [W4]
  Add1/1 -> Add13/1, [W1]
  Add3/1 -> Add14/1, [W3]
  steering motor 2/1(angle) -> Add2/1
  Add2/1 -> Add15/1, [W2]
  From24/1 -> Add4/2
  From26/1 -> Add3/2
  From27/1 -> Add2/2
  From25/1 -> Add1/2
  Pulse Generator/1 -> [B]
  Constant5/1 -> " target steering angle"/2(Xicr)
  " target steering angle"/1(deta4) -> Add12/2
  " target steering angle"/3(deta3) -> Add14/2
  " target steering angle"/2(deta1) -> Add13/2
  " target steering angle"/4(deta2) -> Add15/2
  Input1/1 -> [Yicr]
  [Yicr] -> " target steering angle"/1(Yicr)
  Gain5/1 -> Scope2/1, To Workspace4/1
  Add17/1 -> Gain5/1
  steering motor 4/2(P) -> Add17/1
  steering motor 1/2(P) -> Add17/2
  steering motor 3/2(P) -> Add17/3
  steering motor 2/2(P) -> Add17/4
  Pulse Generator2/1 -> Gain4/1
  Gain4/1 -> [Y]
  Random Number2/1 -> Gain8/1
  Gain8/1 -> [X4]
  Gain9/1 -> [X3]
  Random Number1/1 -> Gain7/1
  Gain6/1 -> [X1]
  Random Number/1 -> Gain6/1
  Gain7/1 -> [X2]
  Random Number3/1 -> Gain9/1
  alpha/1(a1) -> [a1], Bus Creator/1, Variation of the four-wheel slip angles/1
  alpha/4(a4) -> [a4], Bus Creator/4, Variation of the four-wheel slip angles/4
  [u3] -> energy loss caused by lateral slip of wheel/7(u3)
  [nameda1] -> energy loss caused by lateral slip of wheel/1(nameda1)
  [u1] -> energy loss caused by lateral slip of wheel/5(u1)
  [Fx2] -> energy loss caused by lateral slip of wheel/10(Fx2)
  [nameda2] -> energy loss caused by lateral slip of wheel/2(nameda2)
  [Fx4] -> energy loss caused by lateral slip of wheel/12(Fx4)
  [u4] -> energy loss caused by lateral slip of wheel/8(u4)
  [Fx3] -> energy loss caused by lateral slip of wheel/11(Fx3)
  [nameda3] -> energy loss caused by lateral slip of wheel/3(nameda3)
  [nameda4] -> energy loss caused by lateral slip of wheel/4(nameda4)
  [u2] -> energy loss caused by lateral slip of wheel/6(u2)
  [Fx1] -> energy loss caused by lateral slip of wheel/9(Fx1)
  v of the  wheel/2(u2) -> [u2]
  lambda/3(lambda3) -> [nameda3]
  [u1] -> lambda/1(u1)
  v of the  wheel/3(u3) -> [u3]
  [u2] -> lambda/2(u2)
  lambda/4(lambda4) -> [nameda4]
  [W1] -> v of the  wheel/1(deta1)
  [u4] -> lambda/4(u4)
  Constant19/1 -> v of the  wheel/10(B)
  lambda/1(lambda1) -> [nameda1]
  [W2] -> v of the  wheel/2(deta2)
  [Vy] -> v of the  wheel/8(Vy)
  [u3] -> lambda/3(u3)
  [W4] -> v of the  wheel/4(deta4)
  [Vx] -> lambda/5(Vx)
  v of the  wheel/1(u1) -> [u1]
  Constant18/1 -> v of the  wheel/6(lb)
  lambda/2(lambda2) -> [nameda2]
  Constant6/1 -> v of the  wheel/5(la)
  [Vx] -> v of the  wheel/7(Vx)
  [W3] -> v of the  wheel/3(deta3)
  v of the  wheel/4(u4) -> [u4]
  [w] -> v of the  wheel/9(w)
  [a4] -> energy loss by longitudinal slip of wheel/9(a4)
  [Fy4] -> energy loss by longitudinal slip of wheel/4(Fy4)
  Add18/1 -> Integrator5/1
  [Fy3] -> energy loss by longitudinal slip of wheel/3(Fy3)
  energy loss by longitudinal slip of wheel/4(Ph4) -> Add18/4, Scope11/4
  [Fy1] -> energy loss by longitudinal slip of wheel/1(Fy1)
  [Fy2] -> energy loss by longitudinal slip of wheel/2(Fy2)
  energy loss by longitudinal slip of wheel/1(Ph1) -> Scope11/1, Add18/1
  [a1] -> energy loss by longitudinal slip of wheel/6(a1)
  [a3] -> energy loss by longitudinal slip of wheel/8(a3)
  [Vx] -> energy loss by longitudinal slip of wheel/5(Vx)
  energy loss by longitudinal slip of wheel/2(Ph2) -> Scope11/2, Add18/2
  energy loss by longitudinal slip of wheel/3(Ph3) -> Scope11/3, Add18/3
  [a2] -> energy loss by longitudinal slip of wheel/7(a2)
  Abs4/1 -> Integrator3/1
  Integrator7/1 -> Add19/4
  Abs5/1 -> Integrator6/1
  Abs3/1 -> Integrator7/1
  Add19/1 -> [energy]
  Integrator3/1 -> Add19/1
  Abs1/1 -> Integrator4/1
  Integrator4/1 -> Add19/2
  Integrator6/1 -> Add19/3
  energy loss caused by lateral slip of wheel/2(P2) -> Abs1/1
  energy loss caused by lateral slip of wheel/1(P1) -> Abs4/1
  energy loss caused by lateral slip of wheel/3(P3) -> Abs5/1
  energy loss caused by lateral slip of wheel/4(P4) -> Abs3/1
  Constant7/1 -> Total kinetic energy of the wheels/6(r)
  [u2] -> Total kinetic energy of the wheels/2(u2)
  Total kinetic energy of the wheels/1(Ew) -> [Ew]
  [u4] -> Total kinetic energy of the wheels/4(u4)
  [u3] -> Total kinetic energy of the wheels/3(u3)
  [u1] -> Total kinetic energy of the wheels/1(u1)
  Constant8/1 -> Total kinetic energy of the wheels/5(Iw)
  MATLAB Function/1(y) -> Add/1
  Add/1 -> To Workspace3/1, Scope6/1
  [Ew] -> Add/2
  Constant23/1 -> Vx/10(As)
  Constant22/1 -> Vx/9(Cd)
  [Fx3] -> Vx/3(Fx3)
  [m] -> Vx/5(m)
  [Fx2] -> Vx/2(Fx2)
  [Vx] -> Vx/8(vx)
  [Fx1] -> Vx/1(Fx1)
  [Vy] -> Vx/7(Vy)
  [Fx4] -> Vx/4(Fx4)
  [w] -> Vx/6(w)
  Constant9/1 -> "dugoff1 "/1(Fz)
  Constant/1 -> "dugoff1 "/2(u)
  [a1] -> "dugoff1 "/4(alpha1)
  [nameda1] -> "dugoff1 "/3(nameda1)
  [u1] -> "dugoff1 "/5(u1)
  "dugoff1 "/1(f1) -> [f1]
  dugoff2/1(f2) -> [f2]
  [u2] -> dugoff2/5(u2)
  [nameda2] -> dugoff2/3(nameda2)
  [a2] -> dugoff2/4(alpha2)
  Constant20/1 -> dugoff2/2(u)
  Constant21/1 -> dugoff2/1(Fz)
  Constant25/1 -> dugoff3/1(Fz)
  Constant24/1 -> dugoff3/2(u)
  [a3] -> dugoff3/4(alpha3)
  [nameda3] -> dugoff3/3(nameda3)
  [u3] -> dugoff3/5(u3)
  dugoff4/1(f4) -> [f4]
  [u4] -> dugoff4/5(u4)
  [nameda4] -> dugoff4/3(nameda4)
  [a4] -> dugoff4/4(alpha4)
  Constant26/1 -> dugoff4/2(u)
  Constant27/1 -> dugoff4/1(Fz)
  dugoff3/1(f3) -> [f3], Scope9/1
  Integrator5/1 -> Add5/1
  [energy] -> Add5/2
  Add5/1 -> To Workspace2/1, Scope/1
  Pulse Generator5/1 -> [B2]
  Pulse Generator4/1 -> [B4]
  Pulse Generator6/1 -> [B1]
  Pulse Generator7/1 -> [B3]
  [Vy] -> Divide/1
  [Vx] -> Divide/2
  Divide/1 -> Scope4/1
  Bus Creator/1 -> To Workspace/1
  steering motor 4/1(angle) -> Add4/1

== system P_Control/Subsystem/If Action Subsystem ==
  In1 : Inport
  Action Port : ActionPort  ActionPortLabel=if(u1 > 0)
  Input : Outport
  wires:
  In1/1 -> Input/1

== system P_Control/Subsystem/If Action Subsystem1 ==
  In1 : Inport
  Action Port : ActionPort  ActionPortLabel=else
  Out1 : Outport
  wires:
  In1/1 -> Out1/1

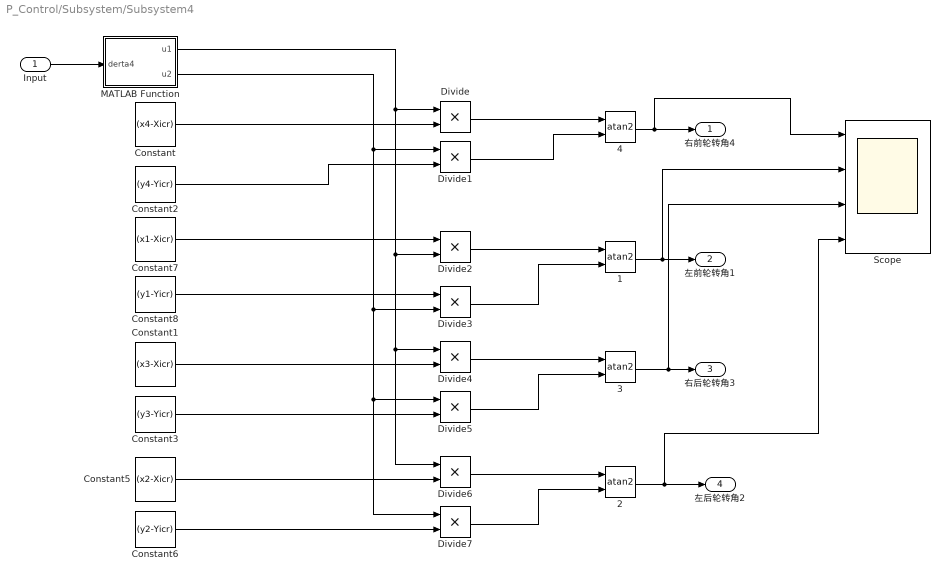
== system P_Control/Subsystem/Subsystem4 ==
  Input : Inport
  {1..4} (4 alike) : Trigonometry  Operator=atan2
  Constant : Constant  Value=(x4-Xicr)
  Constant1 : Constant  Value=(x3-Xicr)
  Constant2 : Constant  Value=(y4-Yicr)
  Constant3 : Constant  Value=(y3-Yicr)
  Constant5 : Constant  Value=(x2-Xicr)
  Constant6 : Constant  Value=(y2-Yicr)
  Constant7 : Constant  Value=(x1-Xicr)
  Constant8 : Constant  Value=(y1-Yicr)
  Divide{,1..7} (8 alike) : Product  Inputs=**
  MATLAB Function : MATLAB Function  TreatAsAtomicUnit=on
  Scope : Scope  NumInputPorts=4
  右前轮转角4 : Outport
  左前轮转角1 : Outport  Port=2
  右后轮转角3 : Outport  Port=3
  左后轮转角2 : Outport  Port=4
  wires:
  2/1 -> 左后轮转角2/1, Scope/4
  Divide7/1 -> 2/2
  Divide6/1 -> 2/1
  Divide5/1 -> 3/2
  Divide4/1 -> 3/1
  3/1 -> 右后轮转角3/1, Scope/3
  MATLAB Function/2(u2) -> Divide1/1, Divide7/1, Divide5/1, Divide3/2
  MATLAB Function/1(u1) -> Divide/1, Divide4/1, Divide6/1, Divide2/2
  Constant/1 -> Divide/2
  1/1 -> 左前轮转角1/1, Scope/2
  Divide3/1 -> 1/2
  Divide2/1 -> 1/1
  Constant8/1 -> Divide3/1
  Constant7/1 -> Divide2/1
  Constant2/1 -> Divide1/2
  Divide1/1 -> 4/2
  Input/1 -> MATLAB Function/1(derta4)
  Divide/1 -> 4/1
  4/1 -> 右前轮转角4/1, Scope/1
  Constant1/1 -> Divide4/2
  Constant3/1 -> Divide5/2
  Constant5/1 -> Divide6/2
  Constant6/1 -> Divide7/2

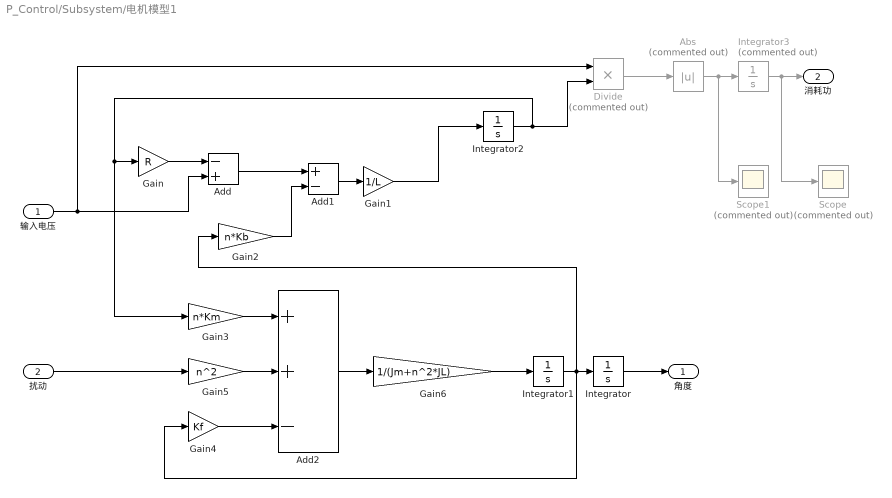
== system P_Control/Subsystem/电机模型1 ==
  输入电压 : Inport
  扰动 : Inport  Port=2
  Abs : Abs  Commented=on  SaturateOnIntegerOverflow=off
  Add : Sum  Inputs=-+
  Add1 : Sum  Inputs=+-
  Add2 : Sum  Inputs=++-
  Divide : Product  Commented=on  Inputs=**
  Gain : Gain  Gain=R
  Gain1 : Gain  Gain=1/L
  Gain2 : Gain  Gain=n*Kb
  Gain3 : Gain  Gain=n*Km
  Gain4 : Gain  Gain=Kf
  Gain5 : Gain  Gain=n^2
  Gain6 : Gain  Gain=1/(Jm+n^2*JL)
  Integrator : Integrator
  Integrator1 : Integrator
  Integrator2 : Integrator  InitialCondition=0.01
  Integrator3 : Integrator  Commented=on
  Scope : Scope  Commented=on
  Scope1 : Scope  Commented=on
  角度 : Outport
  消耗功 : Outport  Port=2
  wires:
  Integrator3/1 -> Scope/1, 消耗功/1
  Abs/1 -> Integrator3/1, Scope1/1
  Divide/1 -> Abs/1
  Gain6/1 -> Integrator1/1
  Add2/1 -> Gain6/1
  Gain4/1 -> Add2/3
  Gain5/1 -> Add2/2
  Gain3/1 -> Add2/1
  扰动/1 -> Gain5/1
  Gain1/1 -> Integrator2/1
  Add1/1 -> Gain1/1
  Gain2/1 -> Add1/2
  Add/1 -> Add1/1
  输入电压/1 -> Add/2, Divide/1
  Gain/1 -> Add/1
  Integrator2/1 -> Divide/2, Gain/1, Gain3/1
  Integrator1/1 -> Integrator/1, Gain4/1, Gain2/1
  Integrator/1 -> 角度/1

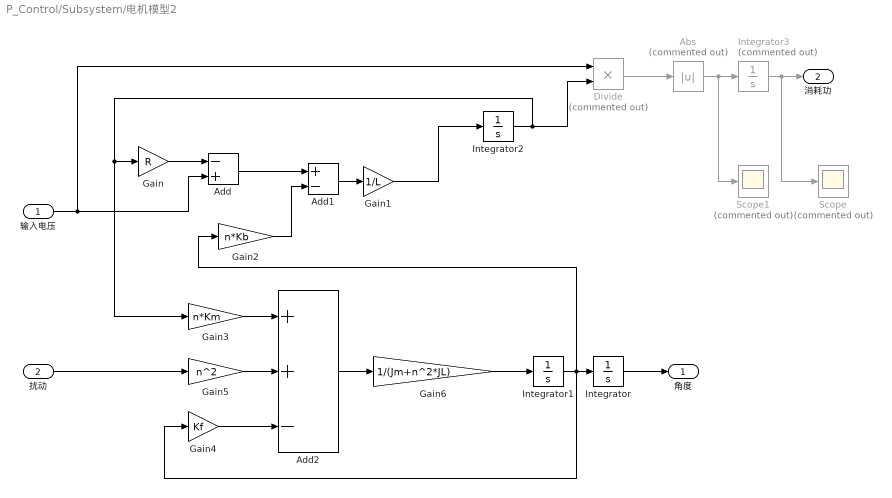
== system P_Control/Subsystem/电机模型2 ==
  输入电压 : Inport
  扰动 : Inport  Port=2
  Abs : Abs  Commented=on  SaturateOnIntegerOverflow=off
  Add : Sum  Inputs=-+
  Add1 : Sum  Inputs=+-
  Add2 : Sum  Inputs=++-
  Divide : Product  Commented=on  Inputs=**
  Gain : Gain  Gain=R
  Gain1 : Gain  Gain=1/L
  Gain2 : Gain  Gain=n*Kb
  Gain3 : Gain  Gain=n*Km
  Gain4 : Gain  Gain=Kf
  Gain5 : Gain  Gain=n^2
  Gain6 : Gain  Gain=1/(Jm+n^2*JL)
  Integrator : Integrator
  Integrator1 : Integrator
  Integrator2 : Integrator  InitialCondition=0.01
  Integrator3 : Integrator  Commented=on
  Scope : Scope  Commented=on
  Scope1 : Scope  Commented=on
  角度 : Outport
  消耗功 : Outport  Port=2
  wires:
  Integrator/1 -> 角度/1
  Integrator1/1 -> Gain2/1, Gain4/1, Integrator/1
  Integrator2/1 -> Gain3/1, Gain/1, Divide/2
  Gain/1 -> Add/1
  输入电压/1 -> Divide/1, Add/2
  Add/1 -> Add1/1
  Gain2/1 -> Add1/2
  Add1/1 -> Gain1/1
  Gain1/1 -> Integrator2/1
  扰动/1 -> Gain5/1
  Gain3/1 -> Add2/1
  Gain5/1 -> Add2/2
  Gain4/1 -> Add2/3
  Add2/1 -> Gain6/1
  Gain6/1 -> Integrator1/1
  Divide/1 -> Abs/1
  Abs/1 -> Scope1/1, Integrator3/1
  Integrator3/1 -> 消耗功/1, Scope/1

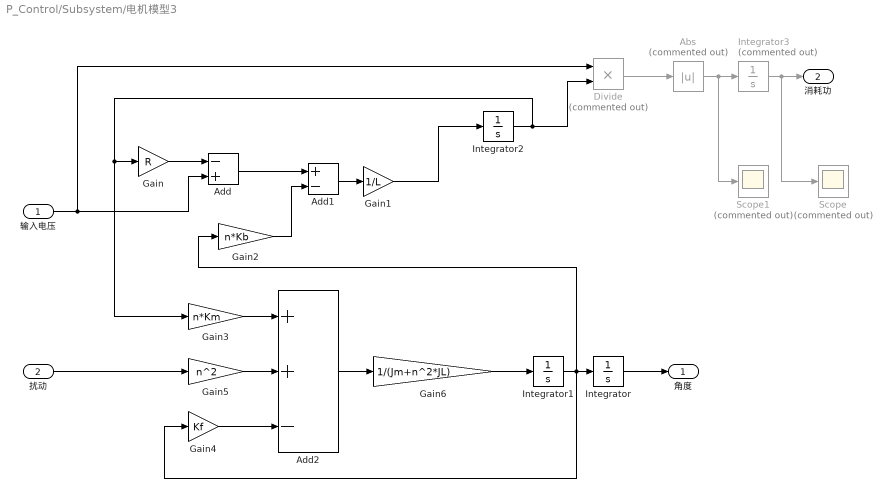
== system P_Control/Subsystem/电机模型3 ==
  输入电压 : Inport
  扰动 : Inport  Port=2
  Abs : Abs  Commented=on  SaturateOnIntegerOverflow=off
  Add : Sum  Inputs=-+
  Add1 : Sum  Inputs=+-
  Add2 : Sum  Inputs=++-
  Divide : Product  Commented=on  Inputs=**
  Gain : Gain  Gain=R
  Gain1 : Gain  Gain=1/L
  Gain2 : Gain  Gain=n*Kb
  Gain3 : Gain  Gain=n*Km
  Gain4 : Gain  Gain=Kf
  Gain5 : Gain  Gain=n^2
  Gain6 : Gain  Gain=1/(Jm+n^2*JL)
  Integrator : Integrator
  Integrator1 : Integrator
  Integrator2 : Integrator  InitialCondition=0.01
  Integrator3 : Integrator  Commented=on
  Scope : Scope  Commented=on
  Scope1 : Scope  Commented=on
  角度 : Outport
  消耗功 : Outport  Port=2
  wires:
  Integrator3/1 -> Scope/1, 消耗功/1
  Abs/1 -> Integrator3/1, Scope1/1
  Divide/1 -> Abs/1
  Gain6/1 -> Integrator1/1
  Add2/1 -> Gain6/1
  Gain4/1 -> Add2/3
  Gain5/1 -> Add2/2
  Gain3/1 -> Add2/1
  扰动/1 -> Gain5/1
  Gain1/1 -> Integrator2/1
  Add1/1 -> Gain1/1
  Gain2/1 -> Add1/2
  Add/1 -> Add1/1
  输入电压/1 -> Add/2, Divide/1
  Gain/1 -> Add/1
  Integrator2/1 -> Divide/2, Gain/1, Gain3/1
  Integrator1/1 -> Integrator/1, Gain4/1, Gain2/1
  Integrator/1 -> 角度/1

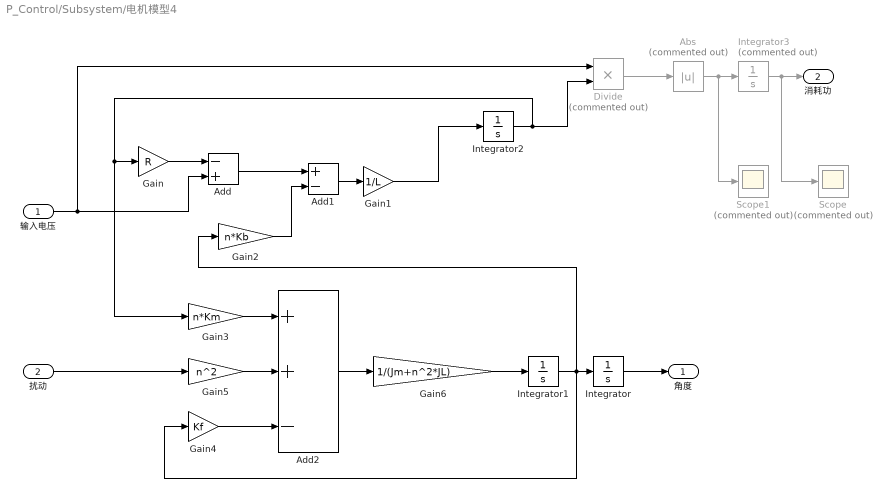
== system P_Control/Subsystem/电机模型4 ==
  输入电压 : Inport
  扰动 : Inport  Port=2
  Abs : Abs  Commented=on  SaturateOnIntegerOverflow=off
  Add : Sum  Inputs=-+
  Add1 : Sum  Inputs=+-
  Add2 : Sum  Inputs=++-
  Divide : Product  Commented=on  Inputs=**
  Gain : Gain  Gain=R
  Gain1 : Gain  Gain=1/L
  Gain2 : Gain  Gain=n*Kb
  Gain3 : Gain  Gain=n*Km
  Gain4 : Gain  Gain=Kf
  Gain5 : Gain  Gain=n^2
  Gain6 : Gain  Gain=1/(Jm+n^2*JL)
  Integrator : Integrator
  Integrator1 : Integrator
  Integrator2 : Integrator  InitialCondition=0.01
  Integrator3 : Integrator  Commented=on
  Scope : Scope  Commented=on
  Scope1 : Scope  Commented=on
  角度 : Outport
  消耗功 : Outport  Port=2
  wires:
  Integrator/1 -> 角度/1
  Integrator1/1 -> Gain2/1, Gain4/1, Integrator/1
  Integrator2/1 -> Gain3/1, Gain/1, Divide/2
  Gain/1 -> Add/1
  输入电压/1 -> Divide/1, Add/2
  Add/1 -> Add1/1
  Gain2/1 -> Add1/2
  Add1/1 -> Gain1/1
  Gain1/1 -> Integrator2/1
  扰动/1 -> Gain5/1
  Gain3/1 -> Add2/1
  Gain5/1 -> Add2/2
  Gain4/1 -> Add2/3
  Add2/1 -> Gain6/1
  Gain6/1 -> Integrator1/1
  Divide/1 -> Abs/1
  Abs/1 -> Scope1/1, Integrator3/1
  Integrator3/1 -> 消耗功/1, Scope/1

== system P_Control/Subsystem/电机模型6 ==
  电流1 : Inport
  干扰 : Inport  Port=2
  Add : Sum
  Add1 : Sum  Inputs=+-
  Add2 : Sum
  Constant : Constant  Value=s_ang3
  Constant1 : Constant  Value=(Jm+n^2*JL)
  Divide : Product  Inputs=*/
  Gain3 : Gain  Gain=n*Km
  Gain4 : Gain  Gain=Kf
  Gain5 : Gain  Gain=n^2
  Integrator : Integrator
  Integrator1 : Integrator
  输出转角 : Outport
  wires:
  Add2/1 -> Divide/1
  Add1/1 -> Add2/2
  Gain5/1 -> Add2/1
  Gain4/1 -> Add1/2
  Gain3/1 -> Add1/1
  Constant1/1 -> Divide/2
  Divide/1 -> Integrator1/1
  Integrator1/1 -> Gain4/1, Integrator/1
  干扰/1 -> Gain5/1
  电流1/1 -> Gain3/1
  Add/1 -> 输出转角/1
  Integrator/1 -> Add/2
  Constant/1 -> Add/1

== system P_Control/Subsystem1/PID1 ==
  e : Inport
  Add : Sum  Inputs=+++
  Derivative : Derivative
  Gain : Gain  Gain=pk
  Gain1 : Gain  Gain=ik
  Gain2 : Gain  Gain=dk
  Integrator : Integrator
  u : Outport
  wires:
  Add/1 -> u/1
  Gain1/1 -> Add/3
  Gain/1 -> Add/2
  Gain2/1 -> Add/1
  Derivative/1 -> Gain2/1
  Integrator/1 -> Gain1/1
  e/1 -> Gain/1, Integrator/1, Derivative/1

== system P_Control/Subsystem1/PID2 ==
  e : Inport
  Add : Sum  Inputs=+++
  Derivative : Derivative
  Gain : Gain  Gain=pd
  Gain1 : Gain  Gain=id
  Gain2 : Gain  Gain=dd
  Integrator : Integrator
  u : Outport
  wires:
  Add/1 -> u/1
  Gain1/1 -> Add/3
  Gain/1 -> Add/2
  Gain2/1 -> Add/1
  Derivative/1 -> Gain2/1
  Integrator/1 -> Gain1/1
  e/1 -> Gain/1, Integrator/1, Derivative/1
